simulink model "pfc_desktop"  (R2024b)
settings: configuration reference "CONFI" (kept outside this file)
InitFcn:
  | fidelity_pfc_vals;
  | Fc=66e3;
values from neighbouring files (symbols this model uses):
  Gs = 2e-2    (= 0.02)    [fidelity_pfc_vals.m]
  s = 1    [fidelity_pfc_vals.m]
  stateSpaceParameters_1 =     [stateSpaceParameters.mat]
  t_ss = tsw/30    (= 5.12820512821e-07)    [fidelity_pfc_vals.m]
  tsw = 1/(fsw*1e3)    (= 1.53846153846e-05)    [fidelity_pfc_vals.m]
undefined symbols (not defined in the file or in its folder): a, b, c, DiscIntNeverNeededParam, Down, Up
libraries: fl_lib x40, nesl_utility x37, ee_lib x11, hdlsllib x7, dspsrcs4 x6, eePwmGenerator x3, hdlssclib x2, spsTriangleGeneratorLib x1, simulink x1
(part 1 of 3)
settings Model: DataDictionary=dic_pfc3ph.sldd  SILPILSystemUnderTest=refmodels  CodeVerificationMode=processor-in-the-loop (pil)  ExtModeTrigDuration=10  Creator=angro  LastModifiedBy=Angel
settings ConfigSetRef: SourceName=CONFI

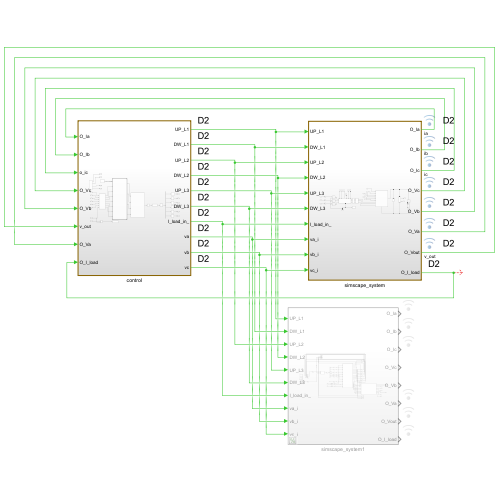
[thumbnail: Simulink's stored preview of the top-level diagram]
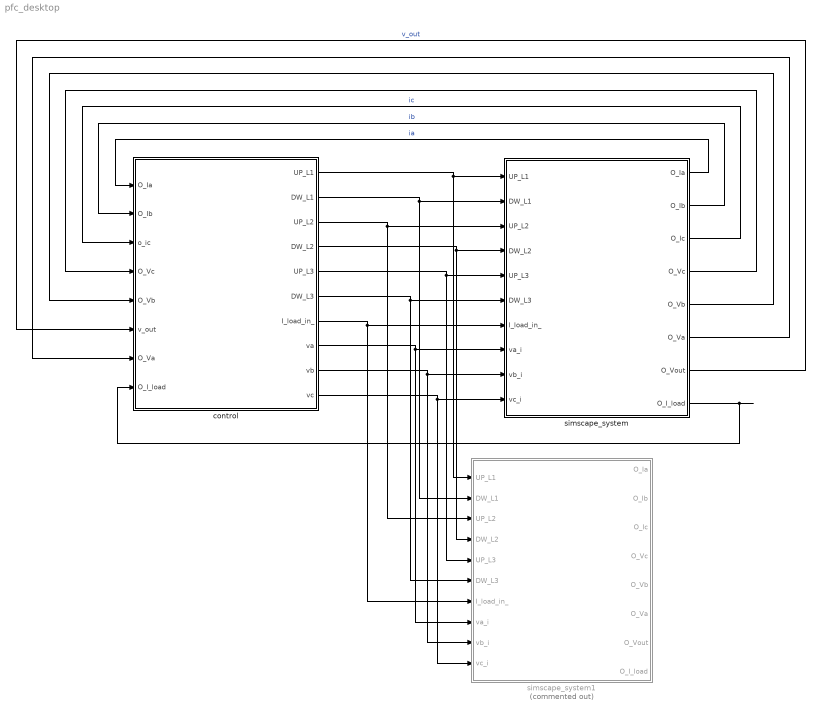
== system pfc_desktop ==
  control : Subsystem
  simscape_system : Subsystem
  simscape_system1 : Subsystem  Commented=on
  wires:
  control/5(UP_L3) -> simscape_system/5(UP_L3), simscape_system1/5(UP_L3)
  control/3(UP_L2) -> simscape_system1/3(UP_L2), simscape_system/3(UP_L2)
  control/1(UP_L1) -> simscape_system1/1(UP_L1), simscape_system/1(UP_L1)
  simscape_system/8(O_I_load) -> control/8(O_I_load)
  control/6(DW_L3) -> simscape_system1/6(DW_L3), simscape_system/6(DW_L3)
  control/4(DW_L2) -> simscape_system1/4(DW_L2), simscape_system/4(DW_L2)
  control/2(DW_L1) -> simscape_system1/2(DW_L1), simscape_system/2(DW_L1)
  control/9(vb) -> simscape_system1/9(vb_i), simscape_system/9(vb_i)
  control/7(I_load_in_) -> simscape_system1/7(I_load_in_), simscape_system/7(I_load_in_)
  control/10(vc) -> simscape_system1/10(vc_i), simscape_system/10(vc_i)
  control/8(va) -> simscape_system1/8(va_i), simscape_system/8(va_i)
  simscape_system/7(O_Vout) -> control/6(v_out)  "v_out"
  simscape_system/1(O_Ia) -> control/1(O_Ia)  "ia"
  simscape_system/2(O_Ib) -> control/2(O_Ib)  "ib"
  simscape_system/3(O_Ic) -> control/3(o_ic)  "ic"
  simscape_system/4(O_Vc) -> control/4(O_Vc)
  simscape_system/5(O_Vb) -> control/5(O_Vb)
  simscape_system/6(O_Va) -> control/7(O_Va)

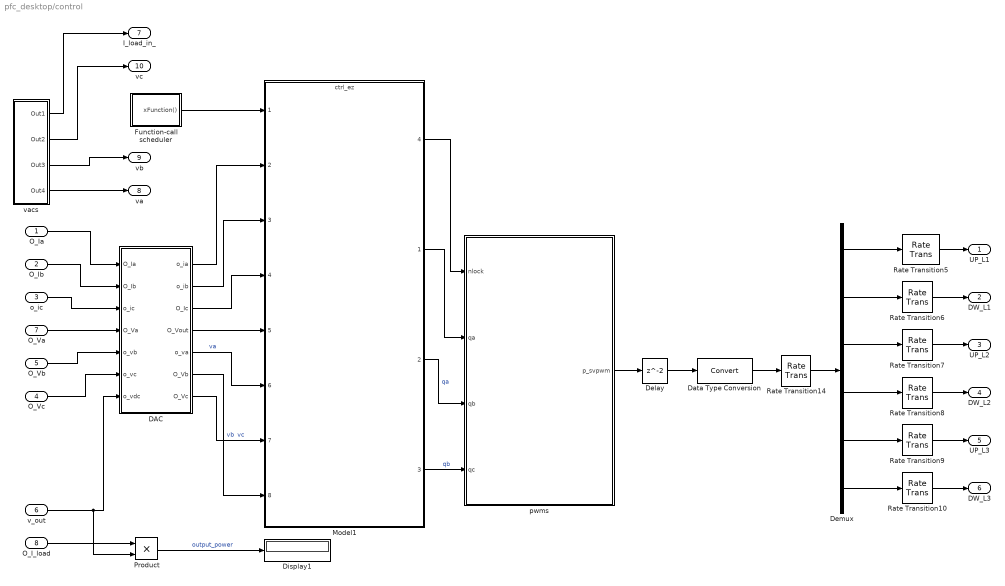
== system pfc_desktop/control ==
  O_Ia : Inport
  O_Ib : Inport  Port=2
  o_ic : Inport  Port=3
  O_Vc : Inport  Port=4
  O_Vb : Inport  Port=5
  v_out : Inport  Port=6
  O_Va : Inport  Port=7
  O_I_load : Inport  Port=8
  DAC : Subsystem
  Data Type Conversion : DataTypeConversion  SaturateOnIntegerOverflow=off  RndMeth=Floor
  Delay : Delay
  Demux : Demux  Outputs=6
  Display1 : Display
  Function-call scheduler : Test Sequence  TreatAsAtomicUnit=on  SystemSampleTime=1/8e3
  Model1 : ModelReference  ModelNameDialog=ctrl_ez.slx  SimulationMode=Normal  ScheduleRates=on  ModelReferenceVersion=1.687
      settings: PortSchema="{\"entries\":[{\"content\":{\"sides\":[{\"content\":{\"connectorIds\":[\"In1\",\"In2\",\"In3\",\"In4\",\"In5\",\"In6\",\"In7\",\"In8\"]},\"type\":\"ConnectorPlacement.EquallySpacedRectSide\",\"uuid\":\"aa3d6869-c98d-43a9-8fec-3792e8050828\"},{\"content\":{\"connectorIds\":[\"Out4\",\"Out1\",\"Out2\",\"Out3\"],\"side\":\"RIGHT\"},\"type\":\"ConnectorPlacement.EquallySpacedRectSide\",\"uuid\":\"39b7aa9e-b1a6-43f6-abd4-8191a6cd49ed\"},{\"content\":{\"side\":\"TOP\"},\"type\":\"ConnectorPlacement.EquallySpacedRectSide\",\"uuid\":\"fc7b43c9-61e3-453d-8da3-63db90188848\"}]},\"type\":\"ConnectorPlacement.EquallySpacedConnector\",\"uuid\":\"b0ed962a-a79f-4d6e-bfe2-e8b5311b0ecd\"}],\"packageUris\":[\"http://schema.mathworks.com/mf0/Connector/R2020b\"],\"version\":\"1.0\"}"
  Product : Product
  Rate Transition{5..10,14} (7 alike) : RateTransition
  pwms : Subsystem
  vacs : Subsystem
  UP_L1 : Outport
  DW_L1 : Outport  Port=2
  UP_L2 : Outport  Port=3
  DW_L2 : Outport  Port=4
  UP_L3 : Outport  Port=5
  DW_L3 : Outport  Port=6
  I_load_in_ : Outport  Port=7
  va : Outport  Port=8
  vb : Outport  Port=9
  vc : Outport  Port=10
  wires:
  Model1/4 -> pwms/1(nlock)
  vacs/3(Out3) -> vb/1
  Model1/1 -> pwms/2(qa)
  vacs/1(Out1) -> I_load_in_/1
  O_I_load/1 -> Product/1
  v_out/1 -> Product/2, DAC/7(o_vdc)
  vacs/4(Out4) -> va/1
  O_Va/1 -> DAC/4(O_Va)
  vacs/2(Out2) -> vc/1
  O_Ia/1 -> DAC/1(O_Ia)
  O_Vc/1 -> DAC/6(o_vc)
  O_Vb/1 -> DAC/5(o_vb)
  O_Ib/1 -> DAC/2(O_Ib)
  o_ic/1 -> DAC/3(o_ic)
  Function-call scheduler/1(xFunction()) -> Model1/1
  DAC/3(O_Ic) -> Model1/4
  DAC/1(o_ia) -> Model1/2
  DAC/2(o_ib) -> Model1/3
  DAC/6(O_Vb) -> Model1/8  "vb"
  DAC/4(O_Vout) -> Model1/5
  Demux/3 -> Rate Transition7/1
  Data Type Conversion/1 -> Rate Transition14/1
  DAC/7(O_Vc) -> Model1/7  "vc"
  DAC/5(o_va) -> Model1/6  "va"
  Product/1 -> Display1/1  "output_power"
  Model1/2 -> pwms/3(qb)  "qa"
  Rate Transition10/1 -> DW_L3/1
  Model1/3 -> pwms/4(qc)  "qb"
  pwms/1(p_svpwm) -> Delay/1
  Demux/6 -> Rate Transition10/1
  Delay/1 -> Data Type Conversion/1
  Rate Transition14/1 -> Demux/1
  Demux/1 -> Rate Transition5/1
  Demux/2 -> Rate Transition6/1
  Demux/4 -> Rate Transition8/1
  Demux/5 -> Rate Transition9/1
  Rate Transition5/1 -> UP_L1/1
  Rate Transition6/1 -> DW_L1/1
  Rate Transition7/1 -> UP_L2/1
  Rate Transition8/1 -> DW_L2/1
  Rate Transition9/1 -> UP_L3/1

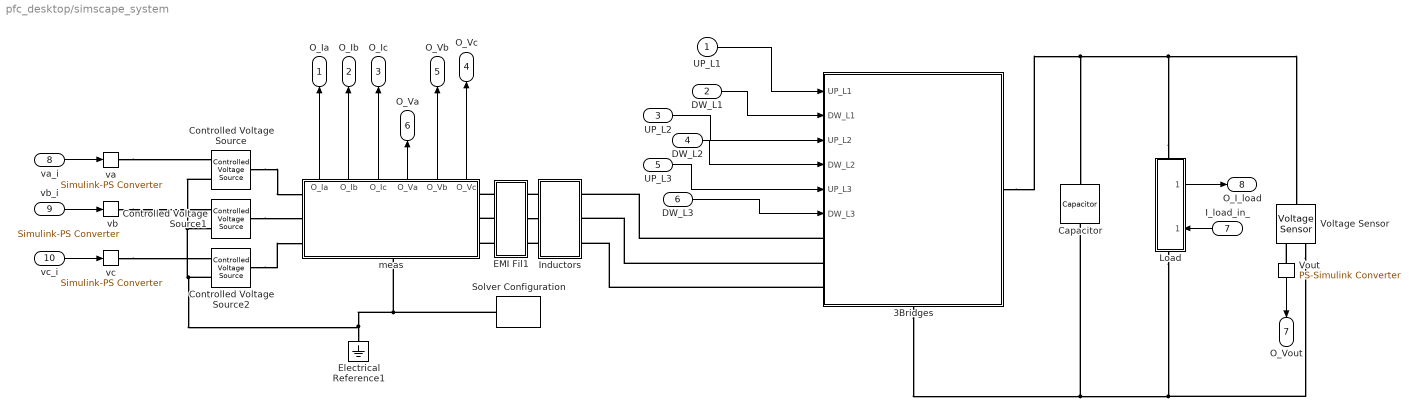
== system pfc_desktop/simscape_system ==
  UP_L1 : Inport
  DW_L1 : Inport  Port=2
  UP_L2 : Inport  Port=3
  DW_L2 : Inport  Port=4
  UP_L3 : Inport  Port=5
  DW_L3 : Inport  Port=6
  I_load_in_ : Inport  Port=7
  va_i : Inport  Port=8
  vb_i : Inport  Port=9
  vc_i : Inport  Port=10
  3Bridges : Subsystem  Variant=on  VariantControlMode=label  VariantControl=3Bridges  LabelModeActiveChoice=Linear FET
      settings: PortSchema="{\"entries\":[{\"content\":{\"sides\":[{\"content\":{\"connectorIds\":[\"In1\",\"In2\",\"In3\",\"In4\",\"In5\",\"In6\",\"LConn1\",\"LConn2\",\"LConn3\"]},\"type\":\"ConnectorPlacement.EquallySpacedRectSide\",\"uuid\":\"8d96b04c-3c8d-475b-959e-eb2713cd0bc4\"},{\"content\":{\"connectorIds\":[\"RConn1\"],\"side\":\"RIGHT\"},\"type\":\"ConnectorPlacement.EquallySpacedRectSide\",\"uuid\":\"f87059ce-ab86-43e3-bcca-ec1681adc212\"},{\"content\":{\"side\":\"TOP\"},\"type\":\"ConnectorPlacement.EquallySpacedRectSide\",\"uuid\":\"b25b4ea6-1654-4766-9c1f-4157e814da22\"},{\"content\":{\"connectorIds\":[\"RConn2\"],\"side\":\"BOTTOM\"},\"type\":\"ConnectorPlacement.EquallySpacedRectSide\",\"uuid\":\"0492bf2a-d02c-4b0c-b7f1-bff02372419b\"}]},\"type\":\"ConnectorPlacement.EquallySpacedConnector\",\"uuid\":\"85107025-6a69-4e99-8d40-1edf872f4d9f\"}],\"packageUris\":[\"http://schema.mathworks.com/mf0/Connector/R2020b\"],\"version\":\"1.0\"}"
  Capacitor : ee_lib/Passive/Capacitor  cap_option=ee.enum.passive.capacitor.capOption.const  c=c_out uF  Cvec=[1e-05, 1e-06] F  Vvec=[0, 10] V  CV_table_symmetry=1  f_vec=[1, 10] kHz  DFext_vec=[.8, 1.2]  enable_C_tol=0  averaging_period=0 s  C_tol=5  tol_distribution=1  nSigma=4  r=1e-3*6 Ohm  g=0 1/Ohm  enable_operating_limits=0  operating_limit_action=2  max_working_voltage_range=[-25, 25] V  power_rating=1 W  maxTemperature=85 degC  thermalEnable=false  thermalMass=1 J/K  fault_action=simscape.enum.assert.action.none  t_fault=1 s  i_specify=off  i_priority=None  i=0 A  i_nominal_specify=off  i_nominal_value=1  i_nominal_unit=A  v_specify=off  v_priority=None  v=0 V  v_nominal_specify=off  v_nominal_value=1  v_nominal_unit=V  vc_specify=on  vc_priority=High  vc=580 V  vc_nominal_specify=off  vc_nominal_value=1  vc_nominal_unit=V  T_specify=off  T_priority=None  T=298.15 K  T_nominal_specify=off  T_nominal_value=1  T_nominal_unit=K
  Controlled Voltage Source : fl_lib/Electrical/Electrical Sources/Controlled Voltage Source
  Controlled Voltage Source1 : fl_lib/Electrical/Electrical Sources/Controlled Voltage Source
  Controlled Voltage Source2 : fl_lib/Electrical/Electrical Sources/Controlled Voltage Source
  EMI Fil1 : Subsystem
  Electrical Reference1 : fl_lib/Electrical/Electrical Elements/Electrical Reference
  Inductors : Subsystem
  Load : Subsystem
      settings: PortSchema="{\"entries\":[{\"content\":{\"sides\":[{\"content\":{\"connectorIds\":[\"LConn1\"]},\"type\":\"ConnectorPlacement.EquallySpacedRectSide\",\"uuid\":\"effb2338-687f-46f5-a36d-064d1cdd1f89\"},{\"content\":{\"connectorIds\":[\"RConn1\"],\"side\":\"RIGHT\"},\"type\":\"ConnectorPlacement.EquallySpacedRectSide\",\"uuid\":\"901d8297-0f3f-4280-ade7-978b42e696ee\"},{\"content\":{\"side\":\"TOP\"},\"type\":\"ConnectorPlacement.EquallySpacedRectSide\",\"uuid\":\"94ece1e5-b3d1-4ff8-a800-be801e6d950f\"},{\"content\":{\"connectorIds\":[\"In1\",\"Out1\"],\"side\":\"BOTTOM\"},\"type\":\"ConnectorPlacement.EquallySpacedRectSide\",\"uuid\":\"36082d89-7906-4f78-be00-891e05fea0eb\"}]},\"type\":\"ConnectorPlacement.EquallySpacedConnector\",\"uuid\":\"9e7f386b-2a06-43cf-bdf5-65e67bd802eb\"}],\"packageUris\":[\"http://schema.mathworks.com/mf0/Connector/R2020b\"],\"version\":\"1.0\"}"
  Solver Configuration : nesl_utility/Solver Configuration  PhysicalDomain=network_engine_domain  SubClassName=solver  LeftPortType=input  RightPortType=generic  Tones=[]  Harmonics=[]  SimulateNoise=off  Profile=off  UseLocalSampling=off  EnableSwitchedLinearOptims=on  FrequencyDomain=off  UseCCode=off  RelTol=0.001  AbsTol=1e-06  MinStep=1e-09  ToWorkspace=off  RevertToSquareIcSolve=off  NumHomotopyIterations=100  PhasorMode=off  PhasorModeNumHarmonics=1  ConsistencySolver=NEWTON_FTOL  IndexReductionMethod=None  DoDC=off  ResidualTolerance=1e-6  ConsistencyTolSource=GLOBAL  ConsistencyAbsTol=0.001  ConsistencyRelTol=0.001  ConsistencyTolFactor=0.001  UseLocalSolver=on  LocalSolverChoice=NE_BACKWARD_EULER_ADVANCER  ResolveIndetEquations=on  FunctionEvalNumThread=1  LocalSolverSampleTime=t_ss  DoFixedCost=on  MaxNonlinIter=1  MaxModeIter=10  ComputeImpulses=off  ImpulseIterations=2  LinearAlgebra=auto  LinearAlgebraNumThread=0  EquationFormulation=NE_TIME_EF  DelaysMemoryBudget=1024  AutomaticFiltering=off  FilteringTimeConstant=0.001  PartitionStorageMethod=EXHAUSTIVE  PartitionMemoryBudget=1024  PartitionMethod=ROBUST  MultibodyUseLocalSolver=off  MultibodyLocalSolverChoice=ODE1  MultibodyLocalSolverSampleTime=0.001
  Voltage Sensor : fl_lib/Electrical/Electrical Sensors/Voltage Sensor
  Vout : nesl_utility/PS-Simulink Converter  PhysicalDomain=network_engine_domain  SubClassName=ps_output  LeftPortType=input  RightPortType=output  PseudoPeriodic=off  Frequencies=[]  VectorFormat=1-D array  Unit=V  AffineConversion=off
  meas : Subsystem
      settings: PortSchema="{\"entries\":[{\"content\":{\"sides\":[{\"content\":{\"connectorIds\":[\"LConn1\",\"LConn2\",\"LConn3\"]},\"type\":\"ConnectorPlacement.EquallySpacedRectSide\",\"uuid\":\"63fb0446-2195-41ce-9f27-949cb83cb3c9\"},{\"content\":{\"connectorIds\":[\"RConn1\",\"RConn2\",\"RConn3\"],\"side\":\"RIGHT\"},\"type\":\"ConnectorPlacement.EquallySpacedRectSide\",\"uuid\":\"9968c418-1dbf-4d06-ba5c-e609e6b84d90\"},{\"content\":{\"connectorIds\":[\"Out1\",\"Out2\",\"Out3\",\"Out4\",\"Out5\",\"Out6\"],\"side\":\"TOP\"},\"type\":\"ConnectorPlacement.EquallySpacedRectSide\",\"uuid\":\"bf7c2fdb-620d-435f-9b2a-06b2c14c987c\"},{\"content\":{\"connectorIds\":[\"RConn4\"],\"side\":\"BOTTOM\"},\"type\":\"ConnectorPlacement.EquallySpacedRectSide\",\"uuid\":\"eb9cce3f-153e-47a2-a171-a4890e03f4a1\"}]},\"type\":\"ConnectorPlacement.EquallySpacedConnector\",\"uuid\":\"4b9ac32f-b167-4dce-a874-653844c6cf4c\"}],\"packageUris\":[\"http://schema.mathworks.com/mf0/Connector/R2020b\"],\"version\":\"1.0\"}"
  va : nesl_utility/Simulink-PS Converter  PhysicalDomain=network_engine_domain  SubClassName=ps_input  LeftPortType=input  RightPortType=output  PseudoPeriodic=off  Frequencies=[]  NoiseDistribution=none  NoiseParameters=[]  Unit=V  AffineConversion=off  FilteringAndDerivatives=zero  SimscapeFilterOrder=1  InputFilterTimeConstant=0.001  UdotUserProvided=0
  vb : nesl_utility/Simulink-PS Converter  PhysicalDomain=network_engine_domain  SubClassName=ps_input  LeftPortType=input  RightPortType=output  PseudoPeriodic=off  Frequencies=[]  NoiseDistribution=none  NoiseParameters=[]  Unit=V  AffineConversion=off  FilteringAndDerivatives=zero  SimscapeFilterOrder=1  InputFilterTimeConstant=0.001  UdotUserProvided=0
  vc : nesl_utility/Simulink-PS Converter  PhysicalDomain=network_engine_domain  SubClassName=ps_input  LeftPortType=input  RightPortType=output  PseudoPeriodic=off  Frequencies=[]  NoiseDistribution=none  NoiseParameters=[]  Unit=V  AffineConversion=off  FilteringAndDerivatives=zero  SimscapeFilterOrder=1  InputFilterTimeConstant=0.001  UdotUserProvided=0
  O_Ia : Outport
  O_Ib : Outport  Port=2
  O_Ic : Outport  Port=3
  O_Vc : Outport  Port=4
  O_Vb : Outport  Port=5
  O_Va : Outport  Port=6
  O_Vout : Outport  Port=7
  O_I_load : Outport  Port=8
  wires:
  Vout/1 -> O_Vout/1
  I_load_in_/1 -> Load/1(I_load_in_)
  meas/1(O_Ia) -> O_Ia/1
  meas/2(O_Ib) -> O_Ib/1
  meas/3(O_Ic) -> O_Ic/1
  meas/6(O_Vc) -> O_Vc/1
  meas/5(O_Vb) -> O_Vb/1
  meas/4(O_Va) -> O_Va/1
  va_i/1 -> va/1
  vb_i/1 -> vb/1
  vc_i/1 -> vc/1
  Load/1(O_I_load) -> O_I_load/1
  UP_L1/1 -> 3Bridges/1(UP_L1)
  DW_L1/1 -> 3Bridges/2(DW_L1)
  UP_L2/1 -> 3Bridges/3(UP_L2)
  DW_L2/1 -> 3Bridges/4(DW_L2)
  UP_L3/1 -> 3Bridges/5(UP_L3)
  DW_L3/1 -> 3Bridges/6(DW_L3)
  connections:
  Controlled Voltage Source/RConn2 -- Solver Configuration/RConn1 -- meas/RConn4 -- Electrical Reference1/LConn1 -- Controlled Voltage Source2/RConn2 -- Controlled Voltage Source1/RConn2
  Inductors/LConn1 -- EMI Fil1/RConn1
  EMI Fil1/RConn2 -- Inductors/LConn2
  Inductors/LConn3 -- EMI Fil1/RConn3
  va/RConn1 -- Controlled Voltage Source/RConn1
  vb/RConn1 -- Controlled Voltage Source1/RConn1
  vc/RConn1 -- Controlled Voltage Source2/RConn1
  Controlled Voltage Source/LConn1 -- meas/LConn1
  Controlled Voltage Source1/LConn1 -- meas/LConn2
  Controlled Voltage Source2/LConn1 -- meas/LConn3
  EMI Fil1/LConn1 -- meas/RConn1
  EMI Fil1/LConn2 -- meas/RConn2
  EMI Fil1/LConn3 -- meas/RConn3
  Load/LConn1 -- 3Bridges/RConn2 -- Capacitor/RConn1 -- Voltage Sensor/RConn2
  Vout/LConn1 -- Voltage Sensor/RConn1
  Load/RConn1 -- Capacitor/LConn1 -- 3Bridges/RConn1 -- Voltage Sensor/LConn1
  3Bridges/LConn1 -- Inductors/RConn1
  3Bridges/LConn2 -- Inductors/RConn2
  3Bridges/LConn3 -- Inductors/RConn3

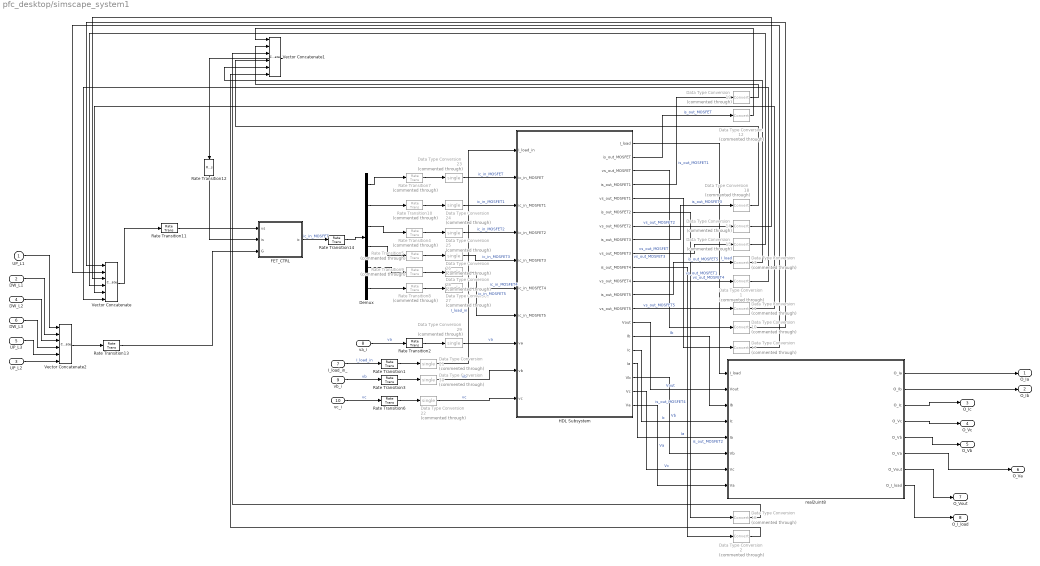
== system pfc_desktop/simscape_system1 ==
  UP_L1 : Inport
  DW_L1 : Inport  Port=2
  UP_L2 : Inport  Port=3
  DW_L2 : Inport  Port=4
  UP_L3 : Inport  Port=5
  DW_L3 : Inport  Port=6
  I_load_in_ : Inport  Port=7  OutDataTypeStr=fixdt(1,18,8)
  va_i : Inport  Port=8  LockScale=on
  vb_i : Inport  Port=9  LockScale=on
  vc_i : Inport  Port=10  LockScale=on
  Data Type Conversion{1..2,10..19} (12 alike) : DataTypeConversion  Commented=through  RndMeth=Nearest  SaturateOnIntegerOverflow=off  LockScale=on
  Data Type Conversion{21..30} (10 alike) : DataTypeConversion  Commented=through  OutDataTypeStr=single  RndMeth=Nearest  SaturateOnIntegerOverflow=off
  Demux : Demux  Outputs=6
  FET_CTRL : Subsystem
  HDL Subsystem : Subsystem
  Rate Transition{1..3,6,11..13} (7 alike) : RateTransition  OutPortSampleTime=t_ss
  Rate Transition{4..5,7..10} (6 alike) : RateTransition  Commented=through  OutPortSampleTime=t_ss
  Rate Transition14 : RateTransition  Integrity=off  OutPortSampleTime=t_ss
  Vector Concatenate : Concatenate  NumInputs=6
  Vector Concatenate1 : Concatenate  NumInputs=6
  Vector Concatenate2 : Concatenate  NumInputs=6
  real2uint8 : Subsystem
  O_Ia : Outport
  O_Ib : Outport  Port=2
  O_Ic : Outport  Port=3
  O_Vc : Outport  Port=4
  O_Vb : Outport  Port=5
  O_Va : Outport  Port=6
  O_Vout : Outport  Port=7
  O_I_load : Outport  Port=8
  wires:
  HDL Subsystem/14(Vout) -> real2uint8/2(Vout)  "Vout"
  HDL Subsystem/13(vs_out_MOSFET5) -> Data Type Conversion11/1  "vs_out_MOSFET5"
  UP_L1/1 -> Vector Concatenate2/1
  HDL Subsystem/16(Ic) -> real2uint8/4(Ic)  "Ic"
  HDL Subsystem/15(Ib) -> real2uint8/3(Ib)  "Ib"
  DW_L1/1 -> Vector Concatenate2/2
  HDL Subsystem/20(Va) -> real2uint8/8(Va)  "Va"
  HDL Subsystem/19(Vc) -> real2uint8/7(Vc)  "Vc"
  DW_L2/1 -> Vector Concatenate2/3
  DW_L3/1 -> Vector Concatenate2/4
  UP_L3/1 -> Vector Concatenate2/5
  HDL Subsystem/18(Vb) -> real2uint8/6(Vb)  "Vb"
  HDL Subsystem/17(Ia) -> real2uint8/5(Ia)  "Ia"
  UP_L2/1 -> Vector Concatenate2/6
  HDL Subsystem/2(is_out_MOSFET) -> Data Type Conversion12/1  "is_out_MOSFET"
  HDL Subsystem/1(I_load) -> real2uint8/1(I_load)  "I_load"
  Vector Concatenate2/1 -> Rate Transition13/1
  FET_CTRL/1(ic) -> Rate Transition14/1  "ic_in_MOSFET"
  I_load_in_/1 -> Rate Transition1/1  "I_load_in"
  Demux/2 -> Rate Transition10/1
  Demux/1 -> Rate Transition7/1
  Rate Transition7/1 -> Data Type Conversion23/1
  va_i/1 -> Rate Transition2/1  "va"
  Demux/4 -> Rate Transition5/1
  Demux/3 -> Rate Transition4/1
  vb_i/1 -> Rate Transition3/1  "vb"
  Demux/6 -> Rate Transition8/1
  Demux/5 -> Rate Transition9/1
  vc_i/1 -> Rate Transition6/1  "vc"
  Rate Transition10/1 -> Data Type Conversion24/1
  Rate Transition4/1 -> Data Type Conversion25/1
  Rate Transition5/1 -> Data Type Conversion26/1
  Data Type Conversion21/1 -> HDL Subsystem/1(I_load_in)  "I_load_in"
  Rate Transition9/1 -> Data Type Conversion28/1
  Rate Transition8/1 -> Data Type Conversion27/1
  Data Type Conversion18/1 -> Vector Concatenate1/4
  Rate Transition2/1 -> Data Type Conversion29/1
  Data Type Conversion24/1 -> HDL Subsystem/3(ic_in_MOSFET1)  "ic_in_MOSFET1"
  Rate Transition1/1 -> Data Type Conversion21/1
  Rate Transition3/1 -> Data Type Conversion30/1
  Data Type Conversion19/1 -> Vector Concatenate1/2
  Rate Transition6/1 -> Data Type Conversion22/1
  Data Type Conversion23/1 -> HDL Subsystem/2(ic_in_MOSFET)  "ic_in_MOSFET"
  Data Type Conversion25/1 -> HDL Subsystem/4(ic_in_MOSFET2)  "ic_in_MOSFET2"
  Data Type Conversion26/1 -> HDL Subsystem/5(ic_in_MOSFET3)  "ic_in_MOSFET3"
  Data Type Conversion28/1 -> HDL Subsystem/7(ic_in_MOSFET5)  "ic_in_MOSFET5"
  Data Type Conversion27/1 -> HDL Subsystem/6(ic_in_MOSFET4)  "ic_in_MOSFET4"
  Data Type Conversion29/1 -> HDL Subsystem/8(va)  "va"
  HDL Subsystem/4(is_out_MOSFET1) -> Data Type Conversion19/1  "is_out_MOSFET1"
  HDL Subsystem/3(vs_out_MOSFET) -> Data Type Conversion10/1  "vs_out_MOSFET"
  Data Type Conversion30/1 -> HDL Subsystem/9(vb)  "vb"
  Data Type Conversion22/1 -> HDL Subsystem/10(vc)  "vc"
  HDL Subsystem/6(is_out_MOSFET2) -> Data Type Conversion16/1  "is_out_MOSFET2"
  HDL Subsystem/5(vs_out_MOSFET1) -> Data Type Conversion17/1  "vs_out_MOSFET1"
  HDL Subsystem/8(is_out_MOSFET3) -> Data Type Conversion18/1  "is_out_MOSFET3"
  HDL Subsystem/7(vs_out_MOSFET2) -> Data Type Conversion14/1  "vs_out_MOSFET2"
  HDL Subsystem/10(is_out_MOSFET4) -> Data Type Conversion2/1  "is_out_MOSFET4"
  HDL Subsystem/9(vs_out_MOSFET3) -> Data Type Conversion15/1  "vs_out_MOSFET3"
  HDL Subsystem/12(is_out_MOSFET5) -> Data Type Conversion13/1  "is_out_MOSFET5"
  HDL Subsystem/11(vs_out_MOSFET4) -> Data Type Conversion1/1  "vs_out_MOSFET4"
  Data Type Conversion12/1 -> Vector Concatenate1/1
  Data Type Conversion14/1 -> Vector Concatenate/3
  Data Type Conversion15/1 -> Vector Concatenate/4
  Data Type Conversion13/1 -> Vector Concatenate1/5
  Data Type Conversion1/1 -> Vector Concatenate/6
  Data Type Conversion11/1 -> Vector Concatenate/5
  Data Type Conversion10/1 -> Vector Concatenate/1
  Data Type Conversion17/1 -> Vector Concatenate/2
  real2uint8/3(O_Ic) -> O_Ic/1
  real2uint8/4(O_Vc) -> O_Vc/1
  real2uint8/5(O_Vb) -> O_Vb/1
  real2uint8/8(O_I_load) -> O_I_load/1
  Data Type Conversion16/1 -> Vector Concatenate1/3
  Data Type Conversion2/1 -> Vector Concatenate1/6
  real2uint8/7(O_Vout) -> O_Vout/1
  Rate Transition13/1 -> FET_CTRL/3(G)
  Vector Concatenate/1 -> Rate Transition11/1
  Vector Concatenate1/1 -> Rate Transition12/1
  Rate Transition14/1 -> Demux/1
  Rate Transition11/1 -> FET_CTRL/1(vs)
  Rate Transition12/1 -> FET_CTRL/2(is)
  real2uint8/1(O_Ia) -> O_Ia/1
  real2uint8/2(O_Ib) -> O_Ib/1
  real2uint8/6(O_Va) -> O_Va/1

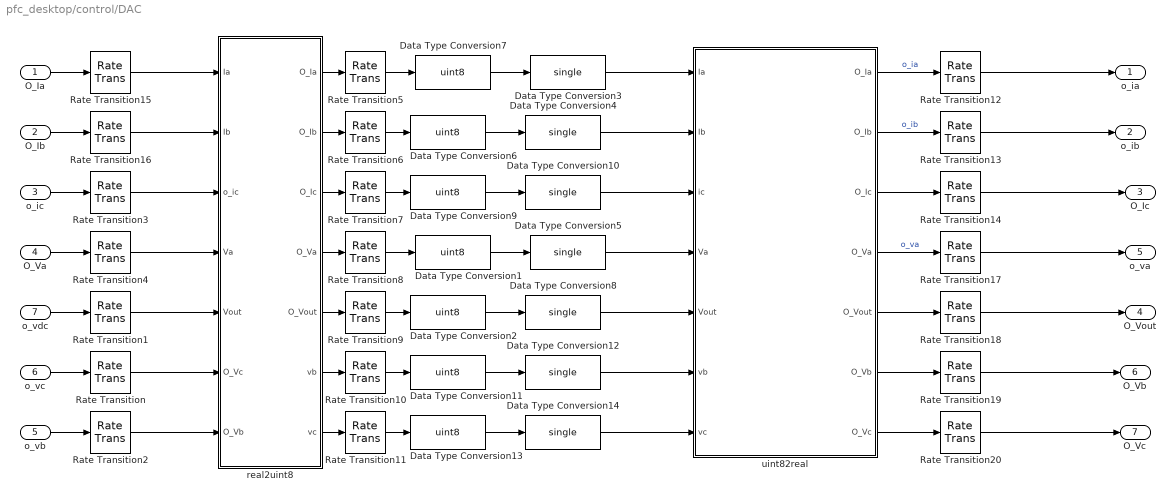
== system pfc_desktop/control/DAC ==
  O_Ia : Inport
  O_Ib : Inport  Port=2
  o_ic : Inport  Port=3
  O_Va : Inport  Port=4
  o_vb : Inport  Port=5
  o_vc : Inport  Port=6
  o_vdc : Inport  Port=7
  Data Type Conversion{1..2,6..7,9,11,13} (7 alike) : DataTypeConversion  OutDataTypeStr=uint8  SaturateOnIntegerOverflow=off  RndMeth=Floor
  Data Type Conversion{3..5,8,10,12,14} (7 alike) : DataTypeConversion  OutDataTypeStr=single  SaturateOnIntegerOverflow=off  RndMeth=Floor
  Rate Transition{,1..4,15..16} (7 alike) : RateTransition  OutPortSampleTime=tsw
  Rate Transition{5..14,17..20} (14 alike) : RateTransition
  real2uint8 : Subsystem
  uint82real : Subsystem
  o_ia : Outport
  o_ib : Outport  Port=2
  O_Ic : Outport  Port=3
  O_Vout : Outport  Port=4
  o_va : Outport  Port=5
  O_Vb : Outport  Port=6
  O_Vc : Outport  Port=7
  wires:
  uint82real/6(O_Vb) -> Rate Transition19/1
  Data Type Conversion7/1 -> Data Type Conversion3/1
  uint82real/4(O_Va) -> Rate Transition17/1  "o_va"
  Data Type Conversion6/1 -> Data Type Conversion4/1
  uint82real/2(O_Ib) -> Rate Transition13/1  "o_ib"
  Data Type Conversion9/1 -> Data Type Conversion10/1
  Data Type Conversion1/1 -> Data Type Conversion5/1
  Data Type Conversion2/1 -> Data Type Conversion8/1
  Data Type Conversion11/1 -> Data Type Conversion12/1
  Data Type Conversion13/1 -> Data Type Conversion14/1
  uint82real/1(O_Ia) -> Rate Transition12/1  "o_ia"
  uint82real/3(O_Ic) -> Rate Transition14/1
  uint82real/5(O_Vout) -> Rate Transition18/1
  uint82real/7(O_Vc) -> Rate Transition20/1
  o_vb/1 -> Rate Transition2/1
  o_vc/1 -> Rate Transition/1
  o_vdc/1 -> Rate Transition1/1
  O_Va/1 -> Rate Transition4/1
  o_ic/1 -> Rate Transition3/1
  O_Ib/1 -> Rate Transition16/1
  O_Ia/1 -> Rate Transition15/1
  Rate Transition4/1 -> real2uint8/4(Va)
  Rate Transition1/1 -> real2uint8/5(Vout)
  Rate Transition/1 -> real2uint8/6(O_Vc)
  Rate Transition2/1 -> real2uint8/7(O_Vb)
  Rate Transition15/1 -> real2uint8/1(Ia)
  Rate Transition16/1 -> real2uint8/2(Ib)
  Rate Transition3/1 -> real2uint8/3(o_ic)
  real2uint8/1(O_Ia) -> Rate Transition5/1
  real2uint8/2(O_Ib) -> Rate Transition6/1
  real2uint8/3(O_Ic) -> Rate Transition7/1
  real2uint8/4(O_Va) -> Rate Transition8/1
  real2uint8/5(O_Vout) -> Rate Transition9/1
  real2uint8/6(vb) -> Rate Transition10/1
  real2uint8/7(vc) -> Rate Transition11/1
  Data Type Conversion5/1 -> uint82real/4(Va)
  Data Type Conversion10/1 -> uint82real/3(ic)
  Data Type Conversion8/1 -> uint82real/5(Vout)
  Data Type Conversion4/1 -> uint82real/2(Ib)
  Data Type Conversion3/1 -> uint82real/1(Ia)
  Data Type Conversion12/1 -> uint82real/6(vb)
  Data Type Conversion14/1 -> uint82real/7(vc)
  Rate Transition5/1 -> Data Type Conversion7/1
  Rate Transition6/1 -> Data Type Conversion6/1
  Rate Transition7/1 -> Data Type Conversion9/1
  Rate Transition8/1 -> Data Type Conversion1/1
  Rate Transition9/1 -> Data Type Conversion2/1
  Rate Transition10/1 -> Data Type Conversion11/1
  Rate Transition11/1 -> Data Type Conversion13/1
  Rate Transition12/1 -> o_ia/1
  Rate Transition13/1 -> o_ib/1
  Rate Transition14/1 -> O_Ic/1
  Rate Transition17/1 -> o_va/1
  Rate Transition18/1 -> O_Vout/1
  Rate Transition19/1 -> O_Vb/1
  Rate Transition20/1 -> O_Vc/1

== system pfc_desktop/control/pwms ==
  nlock : Inport
  qa : Inport  Port=2
  qb : Inport  Port=3
  qc : Inport  Port=4
  EN : Logic  Operator=NOT  IconShape=distinctive  AllPortsSameDT=off  OutDataTypeStr=boolean
  Gain : Gain  Gain=10
  Mux : Mux  Inputs=6
  Rate Transition{1,11..13} (4 alike) : RateTransition
  pwms : Subsystem  Variant=on  VariantControlMode=label  VariantControl=pwms  LabelModeActiveChoice=Subsystem
  p_svpwm : Outport
  wires:
  EN/1 -> Rate Transition1/1  "en_pwm"
  qa/1 -> Rate Transition13/1
  qc/1 -> Rate Transition11/1
  nlock/1 -> EN/1
  qb/1 -> Rate Transition12/1
  Mux/1 -> Gain/1  "p_svpwm"
  Gain/1 -> p_svpwm/1
  Rate Transition13/1 -> pwms/1(qa)
  Rate Transition12/1 -> pwms/2(qb)
  Rate Transition11/1 -> pwms/3(qc)
  pwms/1(UP_L1) -> Mux/1
  pwms/2(DW_L1) -> Mux/2
  pwms/3(UP_L2) -> Mux/3
  pwms/4(DW_L2) -> Mux/4
  pwms/5(UP_L3) -> Mux/5
  pwms/6(DW_L3) -> Mux/6
  Rate Transition1/1 -> pwms/Enable

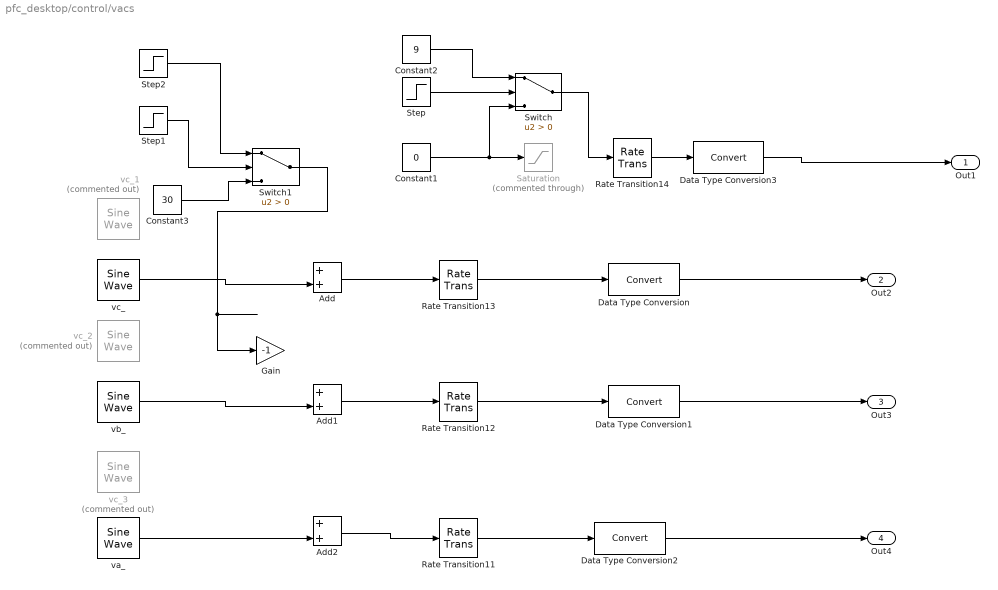
== system pfc_desktop/control/vacs ==
  Add : Sum
  Add1 : Sum
  Add2 : Sum
  Constant1 : Constant  Value=0
  Constant2 : Constant  Value=9
  Constant3 : Constant  Value=30
  Data Type Conversion{,1..3} (4 alike) : DataTypeConversion  SaturateOnIntegerOverflow=off  RndMeth=Floor
  Gain : Gain  Gain=-1
  Rate Transition11 : RateTransition
  Rate Transition12 : RateTransition
  Rate Transition13 : RateTransition
  Rate Transition14 : RateTransition  OutPortSampleTime=t_ss
  Saturation : Saturate  Commented=through  UpperLimit=3
  Step : Step  Time=.3  SampleTime=0
  Step1 : Step  Time=.4345  SampleTime=0
  Step2 : Step  Time=.435  Before=-100  After=0  SampleTime=0
  Switch : Switch  Criteria=u2 > Threshold  SaturateOnIntegerOverflow=off  InputSameDT=off
  Switch1 : Switch  Criteria=u2 > Threshold  SaturateOnIntegerOverflow=off  InputSameDT=off
  va_ : dspsrcs4/Sine Wave  Amplitude=325  Frequency=50  Phase=+pi  SampleMode=Discrete  OutComplex=Real  CompMethod=Table lookup  TableSize=Speed  SampleTime=tsw  SamplesPerFrame=1  ResetState=Restart at time zero  OutputFrames=off  dataType=double  wordLen=16  udDataType=sfix(16)  fracBitsMode=Best precision  numFracBits=15  OutDataTypeStr=double  LastOutDataTypeStr=double
  vb_ : dspsrcs4/Sine Wave  Amplitude=325  Frequency=50  Phase=(-2*pi/3)+pi  SampleMode=Discrete  OutComplex=Real  CompMethod=Table lookup  TableSize=Speed  SampleTime=tsw  SamplesPerFrame=1  ResetState=Restart at time zero  OutputFrames=off  dataType=double  wordLen=16  udDataType=sfix(16)  fracBitsMode=Best precision  numFracBits=15  OutDataTypeStr=double  LastOutDataTypeStr=double
  vc_ : dspsrcs4/Sine Wave  Amplitude=325  Frequency=50  Phase=(2*pi/3)+pi  SampleMode=Discrete  OutComplex=Real  CompMethod=Table lookup  TableSize=Speed  SampleTime=tsw  SamplesPerFrame=1  ResetState=Restart at time zero  OutputFrames=off  dataType=double  wordLen=16  udDataType=sfix(16)  fracBitsMode=Best precision  numFracBits=15  OutDataTypeStr=double  LastOutDataTypeStr=double
  vc_1 : dspsrcs4/Sine Wave  Commented=on  Amplitude=325*.1  Frequency=50*7  Phase=(2*pi/3)+pi  SampleMode=Discrete  OutComplex=Real  CompMethod=Trigonometric fcn  TableSize=Speed  SampleTime=tsw  SamplesPerFrame=1  ResetState=Restart at time zero  OutputFrames=off  dataType=double  wordLen=16  udDataType=sfix(16)  fracBitsMode=Best precision  numFracBits=15  OutDataTypeStr=double  LastOutDataTypeStr=double
  vc_2 : dspsrcs4/Sine Wave  Commented=on  Amplitude=325*.1  Frequency=50*7  Phase=(-2*pi/3)+pi  SampleMode=Discrete  OutComplex=Real  CompMethod=Trigonometric fcn  TableSize=Speed  SampleTime=tsw  SamplesPerFrame=1  ResetState=Restart at time zero  OutputFrames=off  dataType=double  wordLen=16  udDataType=sfix(16)  fracBitsMode=Best precision  numFracBits=15  OutDataTypeStr=double  LastOutDataTypeStr=double
  vc_3 : dspsrcs4/Sine Wave  Commented=on  Amplitude=325*.1  Frequency=50*7  Phase=+pi  SampleMode=Discrete  OutComplex=Real  CompMethod=Trigonometric fcn  TableSize=Speed  SampleTime=tsw  SamplesPerFrame=1  ResetState=Restart at time zero  OutputFrames=off  dataType=double  wordLen=16  udDataType=sfix(16)  fracBitsMode=Best precision  numFracBits=15  OutDataTypeStr=double  LastOutDataTypeStr=double
  Out1 : Outport
  Out2 : Outport  Port=2
  Out3 : Outport  Port=3
  Out4 : Outport  Port=4
  wires:
  vc_/1 -> Add/2
  Rate Transition12/1 -> Data Type Conversion1/1
  Rate Transition13/1 -> Data Type Conversion/1
  Rate Transition11/1 -> Data Type Conversion2/1
  Rate Transition14/1 -> Data Type Conversion3/1
  Step/1 -> Switch/2
  Constant1/1 -> Switch/3, Saturation/1
  Constant2/1 -> Switch/1
  Data Type Conversion/1 -> Out2/1
  Data Type Conversion1/1 -> Out3/1
  Data Type Conversion2/1 -> Out4/1
  Data Type Conversion3/1 -> Out1/1
  Add/1 -> Rate Transition13/1
  vb_/1 -> Add1/2
  va_/1 -> Add2/2
  Add1/1 -> Rate Transition12/1
  Add2/1 -> Rate Transition11/1
  Switch/1 -> Rate Transition14/1
  Step1/1 -> Switch1/2
  Constant3/1 -> Switch1/3
  Step2/1 -> Switch1/1
  Switch1/1 -> Gain/1

== system pfc_desktop/simscape_system/3Bridges ==
  UP_L1 : Inport
  DW_L1 : Inport  Port=2
  UP_L2 : Inport  Port=3
  DW_L2 : Inport  Port=4
  UP_L3 : Inport  Port=5
  DW_L3 : Inport  Port=6
  Linear_FET : Subsystem  VariantControl=Linear FET
  Simscape : Subsystem  VariantControl=Simscape
  L1 : PMIOPort  Side=Left
  L2 : PMIOPort  Port=2  Side=Left
  L3 : PMIOPort  Port=3  Side=Left
  VDC+ : PMIOPort  Port=4  Side=Right
  VDC- : PMIOPort  Port=5  Side=Right

== system pfc_desktop/simscape_system/EMI Fil1 ==
  Coupled Lines (Three-Phase) : ee_lib/Passive/Lines/Coupled Lines (Three-Phase)  prm=1  La=1e-3 H  Lb=1e-3 H  Lc=1e-3 H  L=20 mH  Lmab=3e-4 H  Lmac=3e-4 H  Lmbc=3e-4 H  Lm=0 mH  Ra=0.001 Ohm  Rb=0.001 Ohm  Rc=0.001 Ohm  R=0.001 Ohm  Rm=0 Ohm  Ga=1e-9 1/Ohm  Gb=1e-9 1/Ohm  Gc=1e-9 1/Ohm  G=1e-9 1/Ohm  I_L_specify=off  I_L_priority=High  I_L=[0, 0, 0] A  I_L_nominal_specify=off  I_L_nominal_value=1  I_L_nominal_unit=A  i_La_specify=off  i_La_priority=High  i_La=0 A  i_La_nominal_specify=off  i_La_nominal_value=1  i_La_nominal_unit=A  i_Lb_specify=off  i_Lb_priority=High  i_Lb=0 A  i_Lb_nominal_specify=off  i_Lb_nominal_value=1  i_Lb_nominal_unit=A  i_Lc_specify=off  i_Lc_priority=High  i_Lc=0 A  i_Lc_nominal_specify=off  i_Lc_nominal_value=1  i_Lc_nominal_unit=A
      settings: InternalSimscapePortConfiguration="{\"Bottom\":[],\"Left\":[{\"id\":\"a1\",\"label\":\"a1\",\"type\":\"foundation.electrical.electrical\"},{\"id\":\"b1\",\"label\":\"b1\",\"type\":\"foundation.electrical.electrical\"},{\"id\":\"c1\",\"label\":\"c1\",\"type\":\"foundation.electrical.electrical\"}],\"Right\":[{\"id\":\"a2\",\"label\":\"a2\",\"type\":\"foundation.electrical.electrical\"},{\"id\":\"b2\",\"label\":\"b2\",\"type\":\"foundation.electrical.electrical\"},{\"id\":\"c2\",\"label\":\"c2\",\"type\":\"foundation.electrical.electrical\"}],\"Top\":[]}"
  Resistor : fl_lib/Electrical/Electrical Elements/Resistor  Commented=on  R=10 MOhm  i_specify=off  i_priority=None  i=0 A  i_nominal_specify=off  i_nominal_value=1  i_nominal_unit=A  v_specify=off  v_priority=None  v=0 V  v_nominal_specify=off  v_nominal_value=1  v_nominal_unit=V
  Resistor1 : fl_lib/Electrical/Electrical Elements/Resistor  Commented=on  R=10 MOhm  i_specify=off  i_priority=None  i=0 A  i_nominal_specify=off  i_nominal_value=1  i_nominal_unit=A  v_specify=off  v_priority=None  v=0 V  v_nominal_specify=off  v_nominal_value=1  v_nominal_unit=V
  Resistor2 : fl_lib/Electrical/Electrical Elements/Resistor  Commented=on  R=10 MOhm  i_specify=off  i_priority=None  i=0 A  i_nominal_specify=off  i_nominal_value=1  i_nominal_unit=A  v_specify=off  v_priority=None  v=0 V  v_nominal_specify=off  v_nominal_value=1  v_nominal_unit=V
  +A : PMIOPort  Side=Left
  +B : PMIOPort  Port=2  Side=Left
  +C : PMIOPort  Port=3  Side=Left
  -A : PMIOPort  Port=4  Side=Right
  -B : PMIOPort  Port=5  Side=Right
  -C : PMIOPort  Port=6  Side=Right
  connections:
  Coupled Lines (Three-Phase)/LConn1 -- Resistor2/LConn1 -- +A/RConn1
  +C/RConn1 -- Resistor1/LConn1 -- Coupled Lines (Three-Phase)/LConn3
  -C/RConn1 -- Coupled Lines (Three-Phase)/RConn3
  -B/RConn1 -- Coupled Lines (Three-Phase)/RConn2
  +B/RConn1 -- Coupled Lines (Three-Phase)/LConn2 -- Resistor/LConn1
  -A/RConn1 -- Coupled Lines (Three-Phase)/RConn1
  Resistor1/RConn1 -- Resistor/RConn1 -- Resistor2/RConn1

== system pfc_desktop/simscape_system/Inductors ==
  Inductor1 : ee_lib/Passive/Inductor  l=l_ind uH  enable_L_tol=0  L_tol=0  tol_distribution=1  nSigma=4  r=1e-3 Ohm  g=1e-9 1/Ohm  enable_operating_limits=0  operating_limit_action=2  max_working_current=1 A  power_rating=1 W  fault_action=simscape.enum.assert.action.none  t_fault=1 s  i_L_specify=off  i_L_priority=High  i_L=0 A  i_L_nominal_specify=off  i_L_nominal_value=1  i_L_nominal_unit=A
  Inductor2 : ee_lib/Passive/Inductor  l=l_ind uH  enable_L_tol=0  L_tol=0  tol_distribution=1  nSigma=4  r=1e-3 Ohm  g=1e-9 1/Ohm  enable_operating_limits=0  operating_limit_action=2  max_working_current=1 A  power_rating=1 W  fault_action=simscape.enum.assert.action.none  t_fault=1 s  i_L_specify=off  i_L_priority=High  i_L=0 A  i_L_nominal_specify=off  i_L_nominal_value=1  i_L_nominal_unit=A
  Inductor3 : ee_lib/Passive/Inductor  l=l_ind uH  enable_L_tol=0  L_tol=0  tol_distribution=1  nSigma=4  r=1e-3 Ohm  g=1e-9 1/Ohm  enable_operating_limits=0  operating_limit_action=2  max_working_current=1 A  power_rating=1 W  fault_action=simscape.enum.assert.action.none  t_fault=1 s  i_L_specify=off  i_L_priority=High  i_L=0 A  i_L_nominal_specify=off  i_L_nominal_value=1  i_L_nominal_unit=A
  IAout : PMIOPort  Side=Right
  IA : PMIOPort  Port=2  Side=Left
  Ib : PMIOPort  Port=3  Side=Left
  IBout : PMIOPort  Port=4  Side=Right
  IC : PMIOPort  Port=5  Side=Left
  ICout : PMIOPort  Port=6  Side=Right
  connections:
  Inductor1/LConn1 -- Ib/RConn1
  Inductor1/RConn1 -- IBout/RConn1
  IAout/RConn1 -- Inductor2/RConn1
  Inductor2/LConn1 -- IA/RConn1
  Inductor3/LConn1 -- IC/RConn1
  Inductor3/RConn1 -- ICout/RConn1

== system pfc_desktop/simscape_system/Load ==
  I_load_in_ : Inport
  Controlled Current Source : fl_lib/Electrical/Electrical Sources/Controlled Current Source
  Current Sensor : fl_lib/Electrical/Electrical Sensors/Current Sensor
  I_load : nesl_utility/PS-Simulink Converter  PhysicalDomain=network_engine_domain  SubClassName=ps_output  LeftPortType=input  RightPortType=output  PseudoPeriodic=off  Frequencies=[]  VectorFormat=1-D array  Unit=inherit  AffineConversion=off
  I_load_in : nesl_utility/Simulink-PS Converter  PhysicalDomain=network_engine_domain  SubClassName=ps_input  LeftPortType=input  RightPortType=output  PseudoPeriodic=off  Frequencies=[]  NoiseDistribution=none  NoiseParameters=[]  Unit=1  AffineConversion=off  FilteringAndDerivatives=zero  SimscapeFilterOrder=1  InputFilterTimeConstant=0.001  UdotUserProvided=0
  Iout : PMIOPort  Side=Left
  Iin : PMIOPort  Port=2  Side=Right
  O_I_load : Outport
  wires:
  I_load_in_/1 -> I_load_in/1
  I_load/1 -> O_I_load/1
  connections:
  Current Sensor/LConn1 -- Controlled Current Source/LConn1
  Controlled Current Source/RConn2 -- Iin/RConn1
  I_load_in/RConn1 -- Controlled Current Source/RConn1
  I_load/LConn1 -- Current Sensor/RConn1
  Current Sensor/RConn2 -- Iout/RConn1

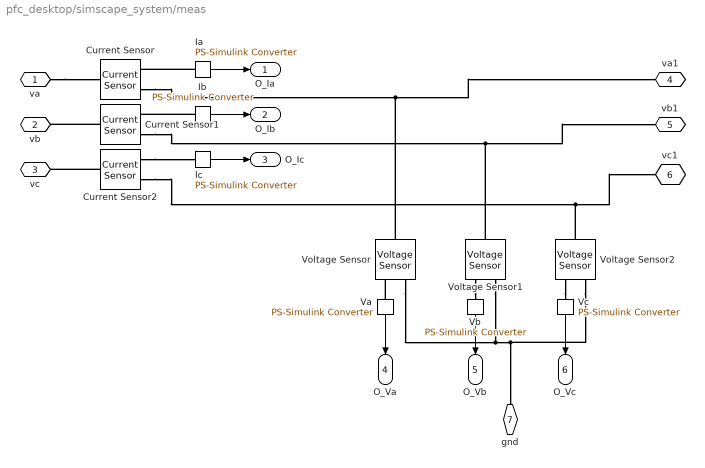
== system pfc_desktop/simscape_system/meas ==
  Current Sensor : fl_lib/Electrical/Electrical Sensors/Current Sensor
  Current Sensor1 : fl_lib/Electrical/Electrical Sensors/Current Sensor
  Current Sensor2 : fl_lib/Electrical/Electrical Sensors/Current Sensor
  Ia : nesl_utility/PS-Simulink Converter  PhysicalDomain=network_engine_domain  SubClassName=ps_output  LeftPortType=input  RightPortType=output  PseudoPeriodic=off  Frequencies=[]  VectorFormat=1-D array  Unit=A  AffineConversion=off
  Ib : nesl_utility/PS-Simulink Converter  PhysicalDomain=network_engine_domain  SubClassName=ps_output  LeftPortType=input  RightPortType=output  PseudoPeriodic=off  Frequencies=[]  VectorFormat=1-D array  Unit=A  AffineConversion=off
  Ic : nesl_utility/PS-Simulink Converter  PhysicalDomain=network_engine_domain  SubClassName=ps_output  LeftPortType=input  RightPortType=output  PseudoPeriodic=off  Frequencies=[]  VectorFormat=1-D array  Unit=A  AffineConversion=off
  Va : nesl_utility/PS-Simulink Converter  PhysicalDomain=network_engine_domain  SubClassName=ps_output  LeftPortType=input  RightPortType=output  PseudoPeriodic=off  Frequencies=[]  VectorFormat=inherit  Unit=inherit  AffineConversion=off
  Vb : nesl_utility/PS-Simulink Converter  PhysicalDomain=network_engine_domain  SubClassName=ps_output  LeftPortType=input  RightPortType=output  PseudoPeriodic=off  Frequencies=[]  VectorFormat=inherit  Unit=inherit  AffineConversion=off
  Vc : nesl_utility/PS-Simulink Converter  PhysicalDomain=network_engine_domain  SubClassName=ps_output  LeftPortType=input  RightPortType=output  PseudoPeriodic=off  Frequencies=[]  VectorFormat=inherit  Unit=inherit  AffineConversion=off
  Voltage Sensor : fl_lib/Electrical/Electrical Sensors/Voltage Sensor
  Voltage Sensor1 : fl_lib/Electrical/Electrical Sensors/Voltage Sensor
  Voltage Sensor2 : fl_lib/Electrical/Electrical Sensors/Voltage Sensor
  va : PMIOPort  Side=Left
  vb : PMIOPort  Port=2  Side=Left
  vc : PMIOPort  Port=3  Side=Left
  va1 : PMIOPort  Port=4  Side=Right
  vb1 : PMIOPort  Port=5  Side=Right
  vc1 : PMIOPort  Port=6  Side=Right
  gnd : PMIOPort  Port=7  Side=Right
  O_Ia : Outport
  O_Ib : Outport  Port=2
  O_Ic : Outport  Port=3
  O_Va : Outport  Port=4
  O_Vb : Outport  Port=5
  O_Vc : Outport  Port=6
  wires:
  Ia/1 -> O_Ia/1
  Ib/1 -> O_Ib/1
  Ic/1 -> O_Ic/1
  Va/1 -> O_Va/1
  Vb/1 -> O_Vb/1
  Vc/1 -> O_Vc/1
  connections:
  va/RConn1 -- Current Sensor/LConn1
  Current Sensor1/LConn1 -- vb/RConn1
  Current Sensor2/LConn1 -- vc/RConn1
  Ia/LConn1 -- Current Sensor/RConn1
  Ib/LConn1 -- Current Sensor1/RConn1
  Current Sensor2/RConn1 -- Ic/LConn1
  Current Sensor/RConn2 -- Voltage Sensor/LConn1 -- va1/RConn1
  Current Sensor1/RConn2 -- Voltage Sensor1/LConn1 -- vb1/RConn1
  Current Sensor2/RConn2 -- Voltage Sensor2/LConn1 -- vc1/RConn1
  Va/LConn1 -- Voltage Sensor/RConn1
  Voltage Sensor/RConn2 -- Voltage Sensor2/RConn2 -- gnd/RConn1 -- Voltage Sensor1/RConn2
  Voltage Sensor1/RConn1 -- Vb/LConn1
  Voltage Sensor2/RConn1 -- Vc/LConn1

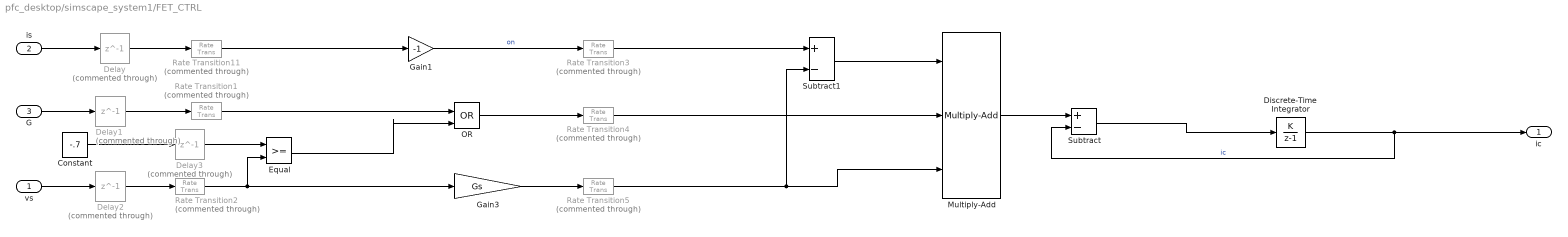
== system pfc_desktop/simscape_system1/FET_CTRL ==
  vs : Inport  OutDataTypeStr=fixdt(1,18,6)  SampleTime=t_ss
  is : Inport  Port=2  OutDataTypeStr=fixdt(1,18,6)  SampleTime=t_ss
  G : Inport  Port=3  SampleTime=t_ss
  Constant : Constant  Value=-.7  OutDataTypeStr=fixdt(1,18,17)  SampleTime=t_ss
  Delay : Delay  Commented=through  DelayLength=1  InputProcessing=Columns as channels (frame based)  SampleTime=t_ss
  Delay1 : Delay  Commented=through  DelayLength=1  InputProcessing=Columns as channels (frame based)  SampleTime=t_ss
  Delay2 : Delay  Commented=through  DelayLength=1  InputProcessing=Columns as channels (frame based)  SampleTime=t_ss
  Delay3 : Delay  Commented=through  DelayLength=1  InitialCondition=-.7  InputProcessing=Columns as channels (frame based)  SampleTime=t_ss
  Discrete-Time Integrator : DiscreteIntegrator  IntegratorMethod=Accumulation: Forward Euler  gainval=1/s  SampleTime=t_ss  OutDataTypeStr=fixdt(1,18,8)  SaturateOnIntegerOverflow=on  LimitOutput=on  UpperSaturationLimit=100  LowerSaturationLimit=-100  ICPrevOutput=DiscIntNeverNeededParam  ICPrevScaledInput=DiscIntNeverNeededParam
  Equal : RelationalOperator  OutDataTypeStr=boolean  RndMeth=Simplest  InputSameDT=off
  Gain1 : Gain  Gain=-1  OutDataTypeStr=fixdt(1,18,12)
  Gain3 : Gain  Gain=Gs  OutDataTypeStr=fixdt(1,18,12)
  Multiply-Add : hdlsllib/HDL Operations/Multiply-Add  Function=c+(a.*b)  datatype=fixdt(1,18,12)  DoSatur=on  FMA=off
  OR : Logic  Operator=OR  IconShape=distinctive  AllPortsSameDT=off  OutDataTypeStr=boolean
  Rate Transition{1..5,11} (6 alike) : RateTransition  Commented=through  OutPortSampleTime=t_ss
  Subtract : Sum  Inputs=+-  OutDataTypeStr=fixdt(1,18,12)
  Subtract1 : Sum  Inputs=+-  OutDataTypeStr=fixdt(1,18,11)
  ic : Outport  SampleTime=t_ss
  wires:
  OR/1 -> Rate Transition4/1
  Subtract1/1 -> Multiply-Add/1
  Gain3/1 -> Rate Transition5/1
  Constant/1 -> Delay3/1
  Equal/1 -> OR/2
  Subtract/1 -> Discrete-Time Integrator/1
  Discrete-Time Integrator/1 -> ic/1, Subtract/2  "ic"
  Gain1/1 -> Rate Transition3/1  "on"
  Multiply-Add/1 -> Subtract/1
  is/1 -> Delay/1
  G/1 -> Delay1/1
  vs/1 -> Delay2/1
  Delay/1 -> Rate Transition11/1
  Delay1/1 -> Rate Transition1/1
  Delay2/1 -> Rate Transition2/1
  Rate Transition11/1 -> Gain1/1
  Rate Transition1/1 -> OR/1
  Rate Transition2/1 -> Gain3/1, Equal/2
  Delay3/1 -> Equal/1
  Rate Transition3/1 -> Subtract1/1
  Rate Transition4/1 -> Multiply-Add/2
  Rate Transition5/1 -> Multiply-Add/3, Subtract1/2

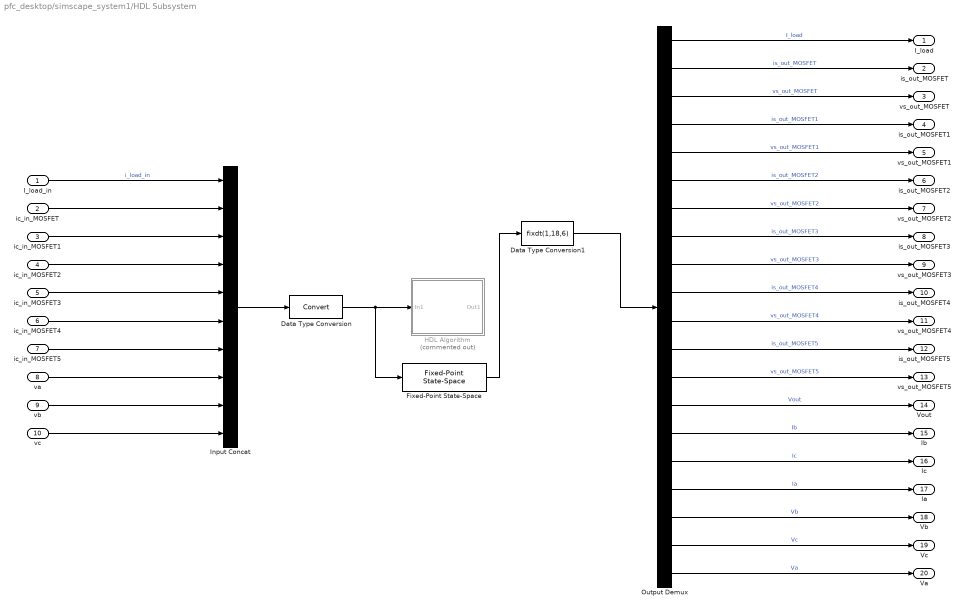
== system pfc_desktop/simscape_system1/HDL Subsystem ==
  I_load_in : Inport  OutDataTypeStr=fixdt(1,18,8)
  ic_in_MOSFET : Inport  Port=2  OutDataTypeStr=fixdt(1,18,8)
  ic_in_MOSFET1 : Inport  Port=3  OutDataTypeStr=fixdt(1,18,8)
  ic_in_MOSFET2 : Inport  Port=4  OutDataTypeStr=fixdt(1,18,8)
  ic_in_MOSFET3 : Inport  Port=5  OutDataTypeStr=fixdt(1,18,8)
  ic_in_MOSFET4 : Inport  Port=6  OutDataTypeStr=fixdt(1,18,8)
  ic_in_MOSFET5 : Inport  Port=7  OutDataTypeStr=fixdt(1,18,8)
  va : Inport  Port=8  OutDataTypeStr=fixdt(1,18,8)
  vb : Inport  Port=9  OutDataTypeStr=fixdt(1,18,8)
  vc : Inport  Port=10  OutDataTypeStr=fixdt(1,18,8)
  Data Type Conversion : DataTypeConversion  SaturateOnIntegerOverflow=off  RndMeth=Floor
  Data Type Conversion1 : DataTypeConversion  OutDataTypeStr=fixdt(1,18,6)  SaturateOnIntegerOverflow=off  RndMeth=Floor
  Fixed-Point State-Space : simulink/Additional Math & Discrete/Additional Discrete/Fixed-Point State-Space  A=fi(stateSpaceParameters_1.Ad,1,25,24)  B=fi(stateSpaceParameters_1.Bd,1,25,31)  C=fi(stateSpaceParameters_1.Cd,1,25,20)  D=fi(stateSpaceParameters_1.Dd,1,25,19)  InitialCondition=fi(stateSpaceParameters_1.X0,1,25,14)  InternalDataType=fixdt(1,25,13)  StateEqScaling=2^0  OutputEqScaling=2^0  DoSatur=off
  HDL Algorithm : Subsystem  Commented=on
  Input Concat : Concatenate  NumInputs=10
  Output Demux : Demux  Outputs=20
  I_load : Outport
  is_out_MOSFET : Outport  Port=2
  vs_out_MOSFET : Outport  Port=3
  is_out_MOSFET1 : Outport  Port=4
  vs_out_MOSFET1 : Outport  Port=5
  is_out_MOSFET2 : Outport  Port=6
  vs_out_MOSFET2 : Outport  Port=7
  is_out_MOSFET3 : Outport  Port=8
  vs_out_MOSFET3 : Outport  Port=9
  is_out_MOSFET4 : Outport  Port=10
  vs_out_MOSFET4 : Outport  Port=11
  is_out_MOSFET5 : Outport  Port=12
  vs_out_MOSFET5 : Outport  Port=13
  Vout : Outport  Port=14
  Ib : Outport  Port=15
  Ic : Outport  Port=16
  Ia : Outport  Port=17
  Vb : Outport  Port=18
  Vc : Outport  Port=19
  Va : Outport  Port=20
  wires:
  Output Demux/7 -> vs_out_MOSFET2/1  "vs_out_MOSFET2"
  Output Demux/2 -> is_out_MOSFET/1  "is_out_MOSFET"
  Output Demux/3 -> vs_out_MOSFET/1  "vs_out_MOSFET"
  Output Demux/4 -> is_out_MOSFET1/1  "is_out_MOSFET1"
  ic_in_MOSFET/1 -> Input Concat/2
  Input Concat/1 -> Data Type Conversion/1
  Output Demux/17 -> Ia/1  "Ia"
  Output Demux/1 -> I_load/1  "I_load"
  vc/1 -> Input Concat/10
  Output Demux/6 -> is_out_MOSFET2/1  "is_out_MOSFET2"
  Output Demux/8 -> is_out_MOSFET3/1  "is_out_MOSFET3"
  Output Demux/15 -> Ib/1  "Ib"
  Output Demux/13 -> vs_out_MOSFET5/1  "vs_out_MOSFET5"
  Output Demux/5 -> vs_out_MOSFET1/1  "vs_out_MOSFET1"
  Output Demux/12 -> is_out_MOSFET5/1  "is_out_MOSFET5"
  Output Demux/10 -> is_out_MOSFET4/1  "is_out_MOSFET4"
  Output Demux/9 -> vs_out_MOSFET3/1  "vs_out_MOSFET3"
  Output Demux/11 -> vs_out_MOSFET4/1  "vs_out_MOSFET4"
  Output Demux/14 -> Vout/1  "Vout"
  Output Demux/16 -> Ic/1  "Ic"
  Output Demux/19 -> Vc/1  "Vc"
  Output Demux/18 -> Vb/1  "Vb"
  Output Demux/20 -> Va/1  "Va"
  vb/1 -> Input Concat/9
  ic_in_MOSFET1/1 -> Input Concat/3
  I_load_in/1 -> Input Concat/1  "i_load_in"
  ic_in_MOSFET3/1 -> Input Concat/5
  ic_in_MOSFET2/1 -> Input Concat/4
  ic_in_MOSFET5/1 -> Input Concat/7
  va/1 -> Input Concat/8
  ic_in_MOSFET4/1 -> Input Concat/6
  Data Type Conversion1/1 -> Output Demux/1
  Data Type Conversion/1 -> Fixed-Point State-Space/1, HDL Algorithm/1(In1)
  Fixed-Point State-Space/1 -> Data Type Conversion1/1

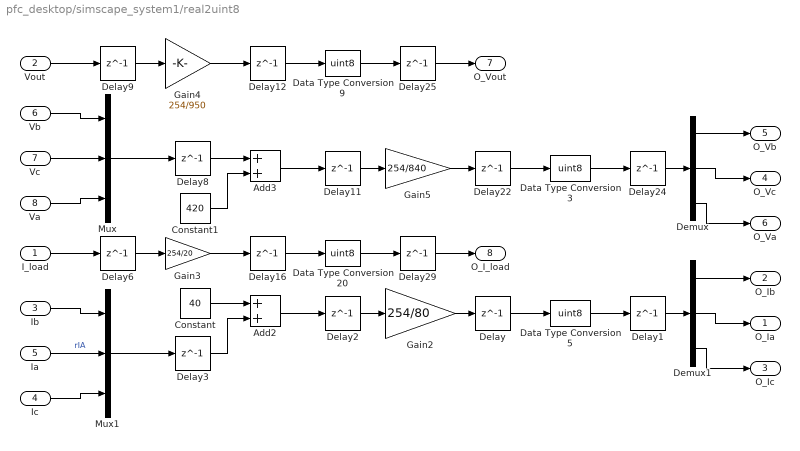
== system pfc_desktop/simscape_system1/real2uint8 ==
  I_load : Inport
  Vout : Inport  Port=2
  Ib : Inport  Port=3
  Ic : Inport  Port=4
  Ia : Inport  Port=5
  Vb : Inport  Port=6
  Vc : Inport  Port=7
  Va : Inport  Port=8
  Add2 : Sum  OutDataTypeStr=Inherit: Same as first input
  Add3 : Sum
  Constant : Constant  Value=40  OutDataTypeStr=fixdt(1,18,6)  SampleTime=-1
  Constant1 : Constant  Value=420  OutDataTypeStr=fixdt(1,18,6)  SampleTime=-1
  Data Type Conversion{3,5,9,20} (4 alike) : DataTypeConversion  OutDataTypeStr=uint8  RndMeth=Nearest  SaturateOnIntegerOverflow=off  LockScale=on
  Delay{,1..3,6,8..9,11..12,16,22,24..25,29} (14 alike) : Delay  DelayLength=1
  Demux : Demux  Outputs=3
  Demux1 : Demux  Outputs=3
  Gain2 : Gain  Gain=254/80  OutDataTypeStr=Inherit: Same as input
  Gain3 : Gain  Gain=254/20  OutDataTypeStr=Inherit: Same as input
  Gain4 : Gain  Gain=254/950  OutDataTypeStr=Inherit: Same as input
  Gain5 : Gain  Gain=254/840  OutDataTypeStr=Inherit: Same as input
  Mux : Mux  Inputs=3
  Mux1 : Mux  Inputs=3
  O_Ia : Outport
  O_Ib : Outport  Port=2
  O_Ic : Outport  Port=3
  O_Vc : Outport  Port=4
  O_Vb : Outport  Port=5
  O_Va : Outport  Port=6
  O_Vout : Outport  Port=7
  O_I_load : Outport  Port=8
  wires:
  Add2/1 -> Delay2/1
  Va/1 -> Mux/3
  Ic/1 -> Mux1/3
  Data Type Conversion9/1 -> Delay25/1
  Vout/1 -> Delay9/1
  Vb/1 -> Mux/1
  Ia/1 -> Mux1/2  "rIA"
  Gain5/1 -> Delay22/1
  Vc/1 -> Mux/2
  Ib/1 -> Mux1/1
  Delay11/1 -> Gain5/1
  I_load/1 -> Delay6/1
  Demux/1 -> O_Vb/1
  Delay29/1 -> O_I_load/1
  Delay9/1 -> Gain4/1
  Mux/1 -> Delay8/1
  Delay6/1 -> Gain3/1
  Mux1/1 -> Delay3/1
  Gain4/1 -> Delay12/1
  Delay2/1 -> Gain2/1
  Delay8/1 -> Add3/1
  Constant1/1 -> Add3/2
  Gain3/1 -> Delay16/1
  Constant/1 -> Add2/1
  Delay3/1 -> Add2/2
  Delay12/1 -> Data Type Conversion9/1
  Add3/1 -> Delay11/1
  Delay16/1 -> Data Type Conversion20/1
  Data Type Conversion20/1 -> Delay29/1
  Delay25/1 -> O_Vout/1
  Gain2/1 -> Delay/1
  Delay22/1 -> Data Type Conversion3/1
  Delay24/1 -> Demux/1
  Delay/1 -> Data Type Conversion5/1
  Data Type Conversion3/1 -> Delay24/1
  Data Type Conversion5/1 -> Delay1/1
  Delay1/1 -> Demux1/1
  Demux/2 -> O_Vc/1
  Demux/3 -> O_Va/1
  Demux1/3 -> O_Ic/1
  Demux1/1 -> O_Ib/1
  Demux1/2 -> O_Ia/1

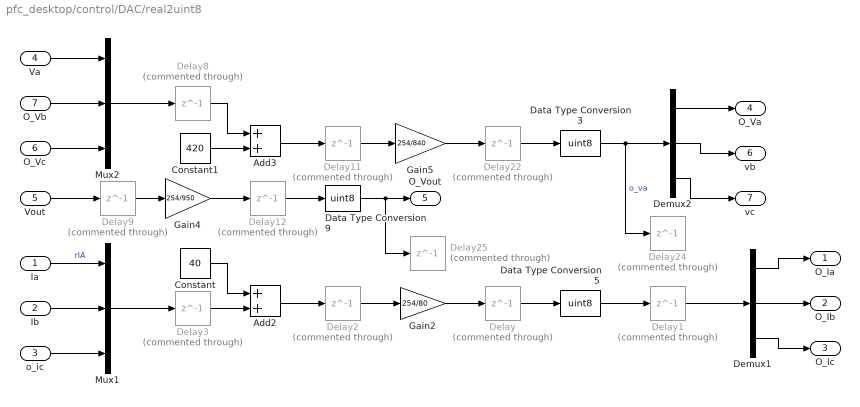
== system pfc_desktop/control/DAC/real2uint8 ==
  Ia : Inport
  Ib : Inport  Port=2
  o_ic : Inport  Port=3
  Va : Inport  Port=4
  Vout : Inport  Port=5
  O_Vc : Inport  Port=6
  O_Vb : Inport  Port=7
  Add2 : Sum  OutDataTypeStr=Inherit: Same as first input
  Add3 : Sum
  Constant : Constant  Value=40  OutDataTypeStr=fixdt(1,18,6)  SampleTime=-1
  Constant1 : Constant  Value=420  OutDataTypeStr=fixdt(1,18,6)  SampleTime=-1
  Data Type Conversion3 : DataTypeConversion  OutDataTypeStr=uint8  RndMeth=Nearest  SaturateOnIntegerOverflow=off  LockScale=on
  Data Type Conversion5 : DataTypeConversion  OutDataTypeStr=uint8  RndMeth=Nearest  SaturateOnIntegerOverflow=off  LockScale=on
  Data Type Conversion9 : DataTypeConversion  OutDataTypeStr=uint8  RndMeth=Nearest  SaturateOnIntegerOverflow=off  LockScale=on
  Delay{,1..3,8..9,11..12,22,24..25} (11 alike) : Delay  Commented=through  DelayLength=1
  Demux1 : Demux  Outputs=3
  Demux2 : Demux  Outputs=3
  Gain2 : Gain  Gain=254/80  OutDataTypeStr=Inherit: Same as input
  Gain4 : Gain  Gain=254/950  OutDataTypeStr=Inherit: Same as input
  Gain5 : Gain  Gain=254/840  OutDataTypeStr=Inherit: Same as input
  Mux1 : Mux  Inputs=3
  Mux2 : Mux  Inputs=3
  O_Ia : Outport
  O_Ib : Outport  Port=2
  O_Ic : Outport  Port=3
  O_Va : Outport  Port=4
  O_Vout : Outport  Port=5
  vb : Outport  Port=6
  vc : Outport  Port=7
  wires:
  Constant/1 -> Add2/1
  Ia/1 -> Mux1/1  "rIA"
  Add2/1 -> Delay2/1
  Add3/1 -> Delay11/1
  Constant1/1 -> Add3/2
  Va/1 -> Mux2/1
  O_Vb/1 -> Mux2/2
  o_ic/1 -> Mux1/3
  O_Vc/1 -> Mux2/3
  Vout/1 -> Delay9/1
  Ib/1 -> Mux1/2
  Mux2/1 -> Delay8/1
  Demux1/2 -> O_Ib/1
  Delay9/1 -> Gain4/1
  Mux1/1 -> Delay3/1
  Demux1/3 -> O_Ic/1
  Delay8/1 -> Add3/1
  Demux2/1 -> O_Va/1
  Gain4/1 -> Delay12/1
  Delay3/1 -> Add2/2
  Delay12/1 -> Data Type Conversion9/1
  Delay11/1 -> Gain5/1
  Data Type Conversion9/1 -> O_Vout/1, Delay25/1
  Delay2/1 -> Gain2/1
  Gain5/1 -> Delay22/1
  Demux2/2 -> vb/1
  Gain2/1 -> Delay/1
  Delay22/1 -> Data Type Conversion3/1
  Delay/1 -> Data Type Conversion5/1
  Delay1/1 -> Demux1/1
  Data Type Conversion3/1 -> Demux2/1, Delay24/1  "o_va"
  Data Type Conversion5/1 -> Delay1/1
  Demux2/3 -> vc/1
  Demux1/1 -> O_Ia/1

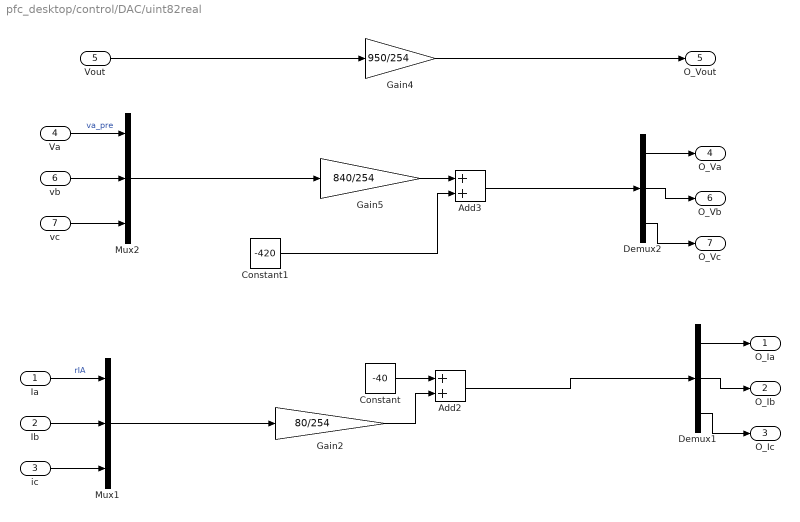
== system pfc_desktop/control/DAC/uint82real ==
  Ia : Inport
  Ib : Inport  Port=2
  ic : Inport  Port=3
  Va : Inport  Port=4
  Vout : Inport  Port=5
  vb : Inport  Port=6
  vc : Inport  Port=7
  Add2 : Sum  OutDataTypeStr=Inherit: Same as first input
  Add3 : Sum
  Constant : Constant  Value=-40  OutDataTypeStr=single  SampleTime=-1
  Constant1 : Constant  Value=-420  OutDataTypeStr=single  SampleTime=-1
  Demux1 : Demux  Outputs=3
  Demux2 : Demux  Outputs=3
  Gain2 : Gain  Gain=80/254  OutDataTypeStr=Inherit: Same as input
  Gain4 : Gain  Gain=950/254  OutDataTypeStr=Inherit: Same as input
  Gain5 : Gain  Gain=840/254  OutDataTypeStr=Inherit: Same as input
  Mux1 : Mux  Inputs=3
  Mux2 : Mux  Inputs=3
  O_Ia : Outport
  O_Ib : Outport  Port=2
  O_Ic : Outport  Port=3
  O_Va : Outport  Port=4
  O_Vout : Outport  Port=5
  O_Vb : Outport  Port=6
  O_Vc : Outport  Port=7
  wires:
  Demux2/1 -> O_Va/1
  Constant1/1 -> Add3/2
  Demux2/3 -> O_Vc/1
  vc/1 -> Mux2/3
  Demux1/2 -> O_Ib/1
  Mux2/1 -> Gain5/1
  vb/1 -> Mux2/2
  Constant/1 -> Add2/1
  Va/1 -> Mux2/1  "va_pre"
  ic/1 -> Mux1/3
  Ib/1 -> Mux1/2
  Ia/1 -> Mux1/1  "rIA"
  Demux1/3 -> O_Ic/1
  Gain2/1 -> Add2/2
  Demux2/2 -> O_Vb/1
  Demux1/1 -> O_Ia/1
  Add3/1 -> Demux2/1
  Add2/1 -> Demux1/1
  Gain4/1 -> O_Vout/1
  Gain5/1 -> Add3/1
  Vout/1 -> Gain4/1
  Mux1/1 -> Gain2/1

== system pfc_desktop/control/pwms/pwms ==
  qa : Inport
  qb : Inport  Port=2
  qc : Inport  Port=3
  Enable : EnablePort
  not_working : Subsystem  VariantControl=pwms
  pwm : Subsystem  VariantControl=Subsystem
  UP_L1 : Outport
  DW_L1 : Outport  Port=2
  UP_L2 : Outport  Port=3
  DW_L2 : Outport  Port=4
  UP_L3 : Outport  Port=5
  DW_L3 : Outport  Port=6
